simulink model "AVR"  (R2018a)
settings: Solver=VariableStepAuto  StartTime=0.0  StopTime=50  RelTol=1e-3
libraries: simulink x1
settings Model: Creator=BIPIN  LastModifiedBy=BIPIN

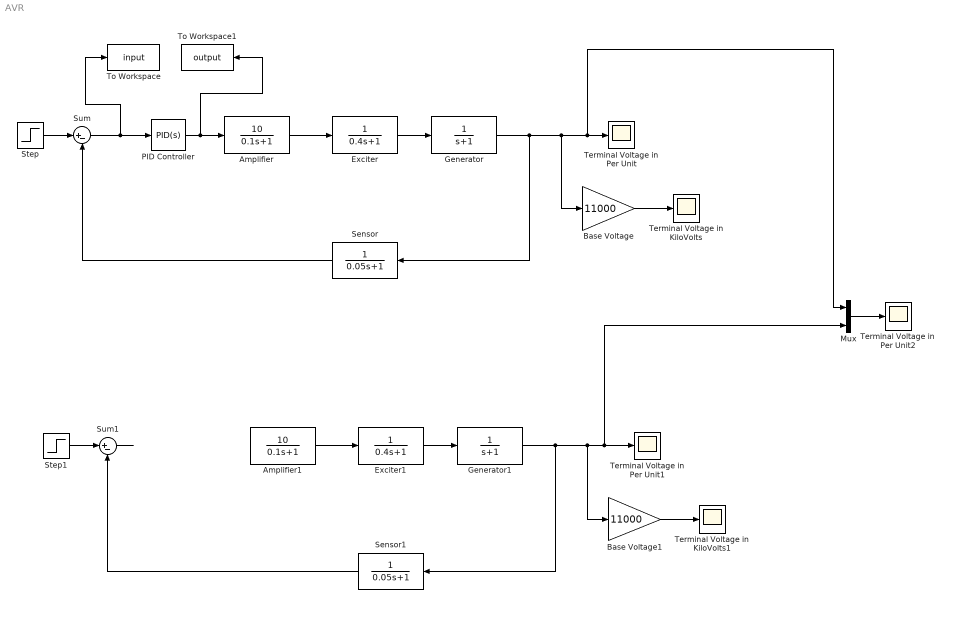
== system AVR ==
  Amplifier : TransferFcn  Numerator=[10]  Denominator=[0.1 1]
  Amplifier1 : TransferFcn  Numerator=[10]  Denominator=[0.1 1]
  Base Voltage : Gain  Gain=11000
  Base Voltage1 : Gain  Gain=11000
  Exciter : TransferFcn  Denominator=[0.4 1]
  Exciter1 : TransferFcn  Denominator=[0.4 1]
  Generator : TransferFcn  Denominator=[1 1]
  Generator1 : TransferFcn  Denominator=[1 1]
  Mux : Mux  Inputs=2
  PID Controller : simulink/Continuous/PID Controller  Controller=PID  TimeDomain=Continuous-time  SampleTime=-1  IntegratorMethod=Forward Euler  FilterMethod=Forward Euler  Form=Parallel  UseFilter=on  ControllerParametersSource=internal  P=1  I=0.25  D=0.2  N=100  InitialConditionSource=internal  InitialConditionForIntegrator=0  InitialConditionForFilter=0  ExternalReset=none  LimitOutput=off  UpperSaturationLimit=inf  LowerSaturationLimit=-inf  LinearizeAsGain=on  AntiWindupMode=none  Kb=1  TrackingMode=off  Kt=1  PParamMin=[]  PParamMax=[]  IParamMin=[]  IParamMax=[]  DParamMin=[]  DParamMax=[]  NParamMin=[]  NParamMax=[]  KbParamMin=[]  KbParamMax=[]  KtParamMin=[]  KtParamMax=[]  POutMin=[]  POutMax=[]  IOutMin=[]  IOutMax=[]  DOutMin=[]  DOutMax=[]  NOutMin=[]  NOutMax=[]  KbOutMin=[]  KbOutMax=[]  KtOutMin=[]  KtOutMax=[]  IntegratorOutMin=[]  IntegratorOutMax=[]  FilterOutMin=[]  FilterOutMax=[]  SumOutMin=[]  SumOutMax=[]  SumI1OutMin=[]  SumI1OutMax=[]  SumI2OutMin=[]  SumI2OutMax=[]  SumI3OutMin=[]  SumI3OutMax=[]  SumDOutMin=[]  SumDOutMax=[]  SaturationOutMin=[]  SaturationOutMax=[]  IntegratorContinuousStateAttributes=''  IntegratorStateMustResolveToSignalObject=off  IntegratorRTWStateStorageClass=Auto  FilterContinuousStateAttributes=''  FilterStateMustResolveToSignalObject=off  FilterRTWStateStorageClass=Auto  DifferentiatorICPrevScaledInput=0  DifferentiatorOutMin=[]  DifferentiatorOutMax=[]  FilterDiffOutCoefMin=[]  FilterDiffOutCoefMax=[]  SumDenOutMin=[]  SumDenOutMax=[]  SumNumOutMin=[]  SumNumOutMax=[]  ReciprocalOutMin=[]  ReciprocalOutMax=[]  DivideOutMin=[]  DivideOutMax=[]  TunerSelectOption=Transfer Function Based (PID Tuner App)
  Sensor : TransferFcn  Denominator=[0.05 1]
  Sensor1 : TransferFcn  Denominator=[0.05 1]
  Step : Step  Time=20  Before=1  SampleTime=0
  Step1 : Step  Time=20  Before=1  SampleTime=0
  Sum : Sum  Inputs=|+-
  Sum1 : Sum  Inputs=|+-
  Terminal Voltage in KiloVolts : Scope
  Terminal Voltage in KiloVolts1 : Scope
  Terminal Voltage in Per Unit : Scope
  Terminal Voltage in Per Unit1 : Scope
  Terminal Voltage in Per Unit2 : Scope
  To Workspace : ToWorkspace  VariableName=input  SampleTime=-1
  To Workspace1 : ToWorkspace  VariableName=output  SampleTime=-1
  wires:
  Step/1 -> Sum/1
  Sum/1 -> To Workspace/1, PID Controller/1
  Amplifier/1 -> Exciter/1
  Exciter/1 -> Generator/1
  Generator/1 -> Sensor/1, Base Voltage/1, Terminal Voltage in Per Unit/1, Mux/1
  Sensor/1 -> Sum/2
  PID Controller/1 -> To Workspace1/1, Amplifier/1
  Base Voltage/1 -> Terminal Voltage in KiloVolts/1
  Sensor1/1 -> Sum1/2
  Amplifier1/1 -> Exciter1/1
  Exciter1/1 -> Generator1/1
  Generator1/1 -> Sensor1/1, Base Voltage1/1, Mux/2, Terminal Voltage in Per Unit1/1
  Base Voltage1/1 -> Terminal Voltage in KiloVolts1/1
  Step1/1 -> Sum1/1
  Mux/1 -> Terminal Voltage in Per Unit2/1
  ? -> Amplifier1/1
  Sum1/1 -> ?
